simulink model "scheme"  (R2017a)
settings: Solver=VariableStepAuto  StartTime=0.0  StopTime=30  RelTol=1e-3
libraries: commanapbnd3 x2, commchan3 x1
settings Model: Creator=Mikle  LastModifiedBy=Mikle

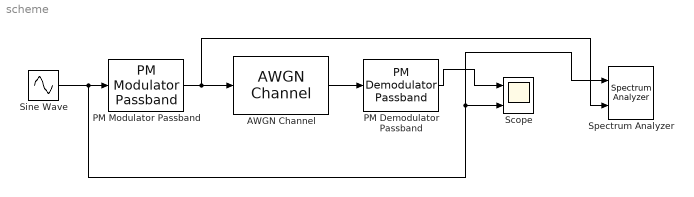
== system scheme ==
  AWGN Channel : commchan3/AWGN Channel  InputProcessing=Columns as channels (frame based)  seed=67  noiseMode="Signal to noise ratio  (Eb/No)"  EbNodB=50  EsNodB=10  SNRdB=10  bitsPerSym=1  Ps=1  Tsym=1  variance=1
  PM Demodulator Passband : commanapbnd3/PM Demodulator Passband  Fc=300  Ph=0  Kc=pi/2  Ho=100
      settings: SourceProductName=Communications System Toolbox  SourceProductBaseCode=CM
  PM Modulator Passband : commanapbnd3/PM Modulator Passband  Fc=300  Ph=0  Kc=pi/2
      settings: SourceProductName=Communications System Toolbox  SourceProductBaseCode=CM
  Scope : Scope  NumInputPorts=2
  Sine Wave : Sin  SineType=Sample based  Samples=3000  SampleTime=0.001
  Spectrum Analyzer : SpectrumAnalyzer  NumInputPorts=2
  wires:
  Sine Wave/1 -> PM Modulator Passband/1, Scope/2, Spectrum Analyzer/1
  PM Demodulator Passband/1 -> Scope/1
  PM Modulator Passband/1 -> Spectrum Analyzer/2, AWGN Channel/1
  AWGN Channel/1 -> PM Demodulator Passband/1
